simulink model "proces"  (R2023a)
settings: Solver=VariableStepAuto  StartTime=0.0  StopTime=10.0  RelTol=1e-3
libraries: MarineRoboticsLib x1
settings Model: Creator=Enio  LastModifiedBy=Enio

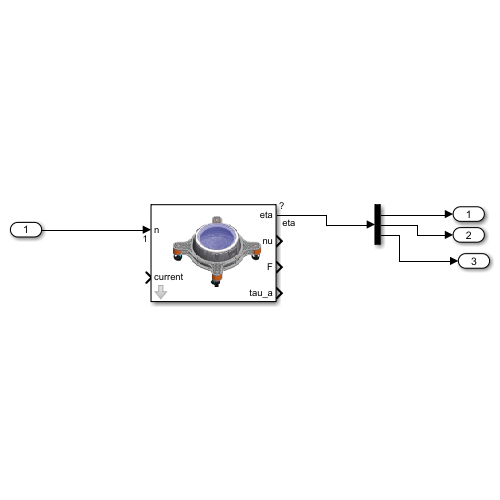
[thumbnail: Simulink's stored preview of the top-level diagram]
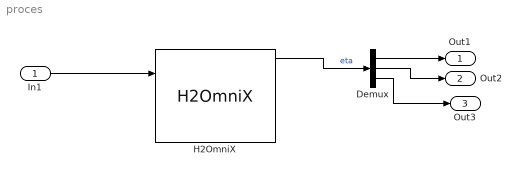
== system proces ==
  In1 : Inport
  Demux : Demux  Outputs=3
  H2OmniX : MarineRoboticsLib/H2OmniX  alpha=[2.1,2.1,0.4]  beta=[1,1,0.24]  betaa=[0,0,0]  nu0=[0,0,0]  eta0=[0,0,0]
  Out1 : Outport
  Out2 : Outport  Port=2
  Out3 : Outport  Port=3
  wires:
  In1/1 -> H2OmniX/1
  H2OmniX/1 -> Demux/1  "eta"
  Demux/1 -> Out1/1
  Demux/2 -> Out2/1
  Demux/3 -> Out3/1
